simulink model "model_10"  (R2021a)
settings: Solver=VariableStepAuto  StartTime=0.0  StopTime=10.0  RelTol=1e-3
libraries: simulink x4
settings Model: Creator=mansi  LastModifiedBy=mansi

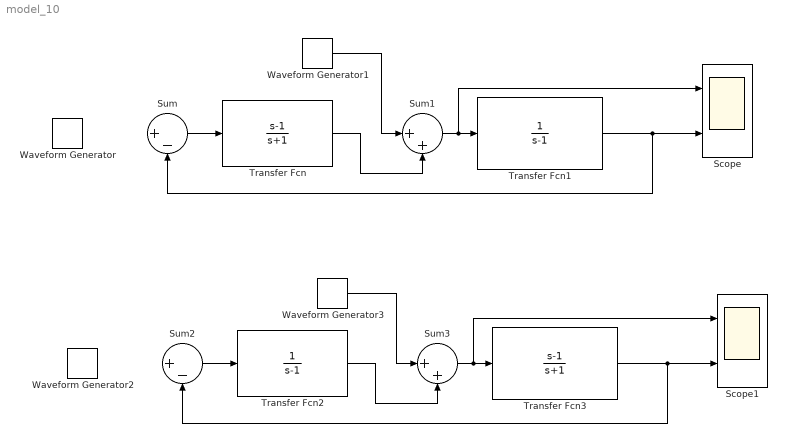
== system model_10 ==
  Scope : Scope  NumInputPorts=2
  Scope1 : Scope  NumInputPorts=2
  Sum : Sum  Inputs=|+-
  Sum1 : Sum  Inputs=|++
  Sum2 : Sum  Inputs=|+-
  Sum3 : Sum  Inputs=|++
  Transfer Fcn : TransferFcn  Numerator=[1,-1]  Denominator=[1 1]
  Transfer Fcn1 : TransferFcn  Denominator=[1,-1]
  Transfer Fcn2 : TransferFcn  Denominator=[1 -1]
  Transfer Fcn3 : TransferFcn  Numerator=[1,-1]  Denominator=[1,1]
  Waveform Generator : simulink/Sources/Waveform Generator  OutMin=[]  OutMax=[]  OutDataTypeStr=double  SelectedSignal=1  Signals=step(0,0,1)  BlockNames=MultiportSwitch_77ad4a2251064ef  SampleTime=0.1
  Waveform Generator1 : simulink/Sources/Waveform Generator  OutMin=[]  OutMax=[]  OutDataTypeStr=double  SelectedSignal=1  Signals=step(0,0,1)  BlockNames=MultiportSwitch_aa92083b733846f  SampleTime=0.1
  Waveform Generator2 : simulink/Sources/Waveform Generator  OutMin=[]  OutMax=[]  OutDataTypeStr=double  SelectedSignal=1  Signals=step(0,0,1)  BlockNames=MultiportSwitch_77ad4a2251064ef  SampleTime=0.1
  Waveform Generator3 : simulink/Sources/Waveform Generator  OutMin=[]  OutMax=[]  OutDataTypeStr=double  SelectedSignal=1  Signals=step(0,0,1)  BlockNames=MultiportSwitch_aa92083b733846f  SampleTime=0.1
  wires:
  Transfer Fcn1/1 -> Sum/2, Scope/2
  Sum/1 -> Transfer Fcn/1
  Transfer Fcn/1 -> Sum1/2
  Sum1/1 -> Scope/1, Transfer Fcn1/1
  Waveform Generator1/1 -> Sum1/1
  Transfer Fcn2/1 -> Sum3/2
  Transfer Fcn3/1 -> Sum2/2, Scope1/2
  Sum3/1 -> Scope1/1, Transfer Fcn3/1
  Sum2/1 -> Transfer Fcn2/1
  Waveform Generator3/1 -> Sum3/1
